simulink library "lib_dGrid"  (R2023b)
settings: Solver=VariableStepAuto  StartTime=0.0  StopTime=10.0  RelTol=1e-3
values from neighbouring files (symbols this model uses):
  C_PM = 10e-3    (= 0.01)    [my_MMC_param.m]
  Cbase = 1/Zbase/wb    (= 3.10849498226e-05)    [my_MMC_param.m]
  f0 = 50/fb    (= 1)    [my_MMC_param.m]
  Fn_filter = 1000    [my_MMC_param.m]
  Fnom = 50    [my_MMC_param.m]
  GFL_APC = 1    [Analysis_Main.m]    (also in initSimu.m; my_MMC_param.m)
  GFL_DVC = 2    [Analysis_Main.m]    (also in initSimu.m; my_MMC_param.m)
  GFM_APC = 3; (values programmed in EMT models)    [Analysis_Main.m]    (also in initSimu.m; my_MMC_param.m = 3)
  GFM_VF = 0    [my_MMC_param.m]
  Ibase = 2*Sbase/(3*Ubase)    [my_MMC_param.m]
  Idcb = Sbase/Udcb    [my_MMC_param.m]
  Ki_Iccsc = 5.15    [my_MMC_param.m]
  Ki_Ireg = CCCTRL.CC.ki    [my_MMC_param.m]
  Ki_Izscc = 100    [my_MMC_param.m]
  Ki_PLL = 1/(CCCTRL.PLL.v0*CCCTRL.PLL.T^2)    [my_MMC_param.m]
  Ki_Preg = 1.0*10    (= 10)    [my_MMC_param.m]
  Ki_Qreg = 1.0*10    (= 10)    [my_MMC_param.m]
  Ki_VAC_GFL = 50    [my_MMC_param.m]
  Ki_VACreg = 10    [my_MMC_param.m]
  Ki_VDCreg = 10    [my_MMC_param.m]
  Ki_WtReg = Kp_WtReg / 0.025    (= 1600)    [my_MMC_param.m]
  Kp_Iccsc = 0.21    [my_MMC_param.m]
  Kp_Ireg = CCCTRL.CC.kp    [my_MMC_param.m]
  Kp_Izscc = 10    [my_MMC_param.m]
  Kp_PLL = 2/CCCTRL.PLL.v0/CCCTRL.PLL.T    [my_MMC_param.m]
  Kp_Preg = 0.5/3*1    (= 0.166666666667)    [my_MMC_param.m]
  Kp_Qreg = 0.5/3*1    (= 0.166666666667)    [my_MMC_param.m]
  Kp_VAC_GFL = 0.5    [my_MMC_param.m]
  Kp_VACreg = 0.01    [my_MMC_param.m]
  Kp_VDCreg = 1    [my_MMC_param.m]
  Kp_WtReg = 40    [my_MMC_param.m]
  Kpv_GFM = 1    [my_MMC_param.m]
  Kpwm = 0.5    [my_MMC_param.m]
  Larm = Larm_pu*(Zbase/wb)    (= 0.0488923985178)    [my_MMC_param.m]
  Lff = Larm_pu/2    (= 0.075)    [my_MMC_param.m]
  Limits_Ireg = [ 2.0  -2.0]    [my_MMC_param.m]
  Limits_Preg = [ 2, -2 ]    [my_MMC_param.m]
  Limits_Qreg = 2*[ 0.42, -0.42 ]    [my_MMC_param.m]
  Limits_VACreg = [ 1.3  -1.3]    [my_MMC_param.m]
  Limits_VDCreg = [ 2.0  -2.0]    [my_MMC_param.m]
  MMC1 = MMC    [Analysis_Main.m]    (also in initSimu.m)
  Nb_PM = 400    [my_MMC_param.m]
  PhaseDelay = 1.0*Ts_Control*2*pi*50    (= 0.0628318530718)    [my_MMC_param.m]
  Pnom = 1000e6    (= 1000000000)    [my_MMC_param.m]
  Rarm = Rarm_pu*Zbase    (= 0.1536)    [my_MMC_param.m]
  Slope_Pref = 0.5    [my_MMC_param.m]
  Slope_Qref = 0.5    [my_MMC_param.m]
  Slope_Vdc_ref = Vnom_dc/2    (= 320000)    [my_MMC_param.m]
  Tdeblock = 1.5    [my_MMC_param.m]
  Ton_CROSSreg = Ton_PQreg+3    (= 7)    [my_MMC_param.m]
  Ton_PQreg = 4    [my_MMC_param.m]
  Ton_VDCreg = 1.5    [my_MMC_param.m]
  Ts = Ts_Control    (= 0.0002)    [my_MMC_param.m]
  Ts_Control = Ts_Power*2    (= 0.0002)    [my_MMC_param.m]
  Ts_Power = 20e-6 * 5    (= 0.0001)    [my_MMC_param.m]
  Ubase = sqrt(2/3)*Vnom_sec    [my_MMC_param.m]
  Udcb = 2*Ubase    [my_MMC_param.m]
  Vc0_PM = 0    [my_MMC_param.m]
  Vnom_dc = 640e3    (= 640000)    [my_MMC_param.m]
  Vnom_sec = 320e3    (= 320000)    [my_MMC_param.m]
  wb = 2*pi*fb    (= 314.159265359)    [my_MMC_param.m]
  Wt_ref_pu = 0.5 * C_PM * (Vnom_dc/Nb_PM)^2 * Nb_PM * 6 / Pnom    (= 0.03072)    [my_MMC_param.m]
undefined symbols (not defined in the file or in its folder): ControlSampleTime, DiscIntNeverNeededParam, MMC, PLL, VSM
libraries: simulink x50, spsCurrentMeasurementLib x20, spsSecondOrderFilterLib x20, spsDiodeLib x12, spsControlledVoltageSourceLib x12, spsSeriesRLCBranchLib x10, spsFirstOrderFilterLib x9, spsVoltageMeasurementLib x8, spsMeanLib x7, FriedrichLibrary x6, $bdroot x6, powerlib_extras x4
(part 7 of 8)

== system lib_dGrid/TL-VSC-configurable control modes/VSC Control/VF mode/PI regulator with anti-windup D1 ==
  note: Anti-windup mechanism: Method of conditionnal integration
      |
      | The integration is suspended if saturation occurs and the
      | control error is of the same sign as the control signal.
      |
      | [1] L.Rundqwist, "Anti-Reset Windup for PID Controllers," Ph.D. Thesis TRFT-1033,
      | Departement of Automatic Control, Lund Institute of Technology, Lund, Sweeden, 1991.
  Error : Inport  SampleTime=Ts
  Compare To Zero : simulink/Logic and Bit Operations/Compare To Zero  relop=>  OutDataTypeStr=uint8  ZeroCross=off
  Compare To Zero1 : simulink/Logic and Bit Operations/Compare To Zero  relop=<  OutDataTypeStr=uint8  ZeroCross=off
  Constant : Constant  Value=0
  Constant1 : Constant  Value=UpperLimit
  Constant3 : Constant  Value=LowerLimit
  Discrete-Time Integrator : DiscreteIntegrator  IntegratorMethod=Integration: Trapezoidal  InitialCondition=Init  SampleTime=Ts  LimitOutput=on  UpperSaturationLimit=UpperLimit  LowerSaturationLimit=LowerLimit  ShowStatePort=on  ICPrevOutput=DiscIntNeverNeededParam  ICPrevScaledInput=DiscIntNeverNeededParam
  Kp4 : Gain  Gain=Kp  SaturateOnIntegerOverflow=on  SampleTime=Ts  OutDataTypeStr=Inherit: Same as input  ParamDataTypeStr=Inherit: Same as input
  Kp5 : Gain  Gain=Ki  SaturateOnIntegerOverflow=on  SampleTime=Ts  OutDataTypeStr=Inherit: Same as input  ParamDataTypeStr=Inherit: Same as input
  Logical Operator : Logic  AllPortsSameDT=off  OutDataTypeStr=boolean
  Logical Operator1 : Logic  AllPortsSameDT=off  OutDataTypeStr=boolean
  Logical Operator2 : Logic  Operator=OR  AllPortsSameDT=off  OutDataTypeStr=boolean
  Relational Operator : RelationalOperator  OutDataTypeStr=boolean  InputSameDT=off
  Relational Operator1 : RelationalOperator  Operator=<=  OutDataTypeStr=boolean  InputSameDT=off
  Saturation2 : Saturate  UpperLimit=UpperLimit  LowerLimit=LowerLimit  SampleTime=Ts
  Sum1 : Sum  InputSameDT=on  SaturateOnIntegerOverflow=on  SampleTime=Ts  OutDataTypeStr=Inherit: Same as first input
  Sum6 : Sum  InputSameDT=on  SaturateOnIntegerOverflow=on  SampleTime=Ts  OutDataTypeStr=Inherit: Same as first input
  Switch : Switch  Criteria=u2 > Threshold  SaturateOnIntegerOverflow=off  InputSameDT=off
  Zero-Order Hold : ZeroOrderHold  SampleTime=Ts
  Out : Outport  SampleTime=Ts  InitialOutput=0  VectorParamsAs1DForOutWhenUnconnected=off
  wires:
  Kp5/1 -> Switch/3
  Switch/1 -> Discrete-Time Integrator/1
  Saturation2/1 -> Out/1
  Discrete-Time Integrator/1 -> Sum6/2
  Kp4/1 -> Zero-Order Hold/1
  Sum6/1 -> Saturation2/1
  Error/1 -> Kp5/1, Kp4/1, Compare To Zero/1, Compare To Zero1/1
  Compare To Zero1/1 -> Logical Operator1/2  "Error_is_negative"
  Logical Operator1/1 -> Logical Operator2/2
  Logical Operator/1 -> Logical Operator2/1
  Compare To Zero/1 -> Logical Operator/2  "Error_is_positive"
  Constant3/1 -> Relational Operator1/2
  Constant1/1 -> Relational Operator/2
  Relational Operator1/1 -> Logical Operator1/1  "LowerLimit_Is_Reached"
  Relational Operator/1 -> Logical Operator/1  "UpperLimit_is_Reached"
  Logical Operator2/1 -> Switch/2
  Sum1/1 -> Relational Operator/1, Relational Operator1/1
  Discrete-Time Integrator/State -> Sum1/1
  Zero-Order Hold/1 -> Sum6/1, Sum1/2
  Constant/1 -> Switch/1

== system lib_dGrid/TL-VSC-configurable control modes/VSC Control/VF mode/PI regulator with anti-windup D2 ==
  note: Anti-windup mechanism: Method of conditionnal integration
      |
      | The integration is suspended if saturation occurs and the
      | control error is of the same sign as the control signal.
      |
      | [1] L.Rundqwist, "Anti-Reset Windup for PID Controllers," Ph.D. Thesis TRFT-1033,
      | Departement of Automatic Control, Lund Institute of Technology, Lund, Sweeden, 1991.
  Error : Inport  SampleTime=Ts
  Compare To Zero : simulink/Logic and Bit Operations/Compare To Zero  relop=>  OutDataTypeStr=uint8  ZeroCross=off
  Compare To Zero1 : simulink/Logic and Bit Operations/Compare To Zero  relop=<  OutDataTypeStr=uint8  ZeroCross=off
  Constant : Constant  Value=0
  Constant1 : Constant  Value=UpperLimit
  Constant3 : Constant  Value=LowerLimit
  Discrete-Time Integrator : DiscreteIntegrator  IntegratorMethod=Integration: Trapezoidal  InitialCondition=Init  SampleTime=Ts  LimitOutput=on  UpperSaturationLimit=UpperLimit  LowerSaturationLimit=LowerLimit  ShowStatePort=on  ICPrevOutput=DiscIntNeverNeededParam  ICPrevScaledInput=DiscIntNeverNeededParam
  Kp4 : Gain  Gain=Kp  SaturateOnIntegerOverflow=on  SampleTime=Ts  OutDataTypeStr=Inherit: Same as input  ParamDataTypeStr=Inherit: Same as input
  Kp5 : Gain  Gain=Ki  SaturateOnIntegerOverflow=on  SampleTime=Ts  OutDataTypeStr=Inherit: Same as input  ParamDataTypeStr=Inherit: Same as input
  Logical Operator : Logic  AllPortsSameDT=off  OutDataTypeStr=boolean
  Logical Operator1 : Logic  AllPortsSameDT=off  OutDataTypeStr=boolean
  Logical Operator2 : Logic  Operator=OR  AllPortsSameDT=off  OutDataTypeStr=boolean
  Relational Operator : RelationalOperator  OutDataTypeStr=boolean  InputSameDT=off
  Relational Operator1 : RelationalOperator  Operator=<=  OutDataTypeStr=boolean  InputSameDT=off
  Saturation2 : Saturate  UpperLimit=UpperLimit  LowerLimit=LowerLimit  SampleTime=Ts
  Sum1 : Sum  InputSameDT=on  SaturateOnIntegerOverflow=on  SampleTime=Ts  OutDataTypeStr=Inherit: Same as first input
  Sum6 : Sum  InputSameDT=on  SaturateOnIntegerOverflow=on  SampleTime=Ts  OutDataTypeStr=Inherit: Same as first input
  Switch : Switch  Criteria=u2 > Threshold  SaturateOnIntegerOverflow=off  InputSameDT=off
  Zero-Order Hold : ZeroOrderHold  SampleTime=Ts
  Out : Outport  SampleTime=Ts  InitialOutput=0  VectorParamsAs1DForOutWhenUnconnected=off
  wires:
  Kp5/1 -> Switch/3
  Switch/1 -> Discrete-Time Integrator/1
  Saturation2/1 -> Out/1
  Discrete-Time Integrator/1 -> Sum6/2
  Kp4/1 -> Zero-Order Hold/1
  Sum6/1 -> Saturation2/1
  Error/1 -> Kp5/1, Kp4/1, Compare To Zero/1, Compare To Zero1/1
  Compare To Zero1/1 -> Logical Operator1/2  "Error_is_negative"
  Logical Operator1/1 -> Logical Operator2/2
  Logical Operator/1 -> Logical Operator2/1
  Compare To Zero/1 -> Logical Operator/2  "Error_is_positive"
  Constant3/1 -> Relational Operator1/2
  Constant1/1 -> Relational Operator/2
  Relational Operator1/1 -> Logical Operator1/1  "LowerLimit_Is_Reached"
  Relational Operator/1 -> Logical Operator/1  "UpperLimit_is_Reached"
  Logical Operator2/1 -> Switch/2
  Sum1/1 -> Relational Operator/1, Relational Operator1/1
  Discrete-Time Integrator/State -> Sum1/1
  Zero-Order Hold/1 -> Sum6/1, Sum1/2
  Constant/1 -> Switch/1

== system lib_dGrid/TL-VSC-configurable control modes/VSC Control/VSM Control/DQ damping1 Need New paras or New implementation ==
  enable_damp_dq : Inport
  u_dq0 : Inport  Port=2
  Gain2 : Gain  Gain=OmLead
  Gain5 : Gain  Gain=OmLag
  Integrator (inertia) : DiscreteIntegrator  IntegratorMethod=Integration: Backward Euler  gainval=1  InitialCondition=1  SampleTime=ControlSampleTime  ICPrevOutput=DiscIntNeverNeededParam  ICPrevScaledInput=DiscIntNeverNeededParam
  Product : Product
  Product1 : Product
  Sum : Sum  Inputs=|+-
  Sum2 : Sum  Inputs=++|
  Zero-Order Hold : ZeroOrderHold  SampleTime=Ts
  damp_dq0 : Outport  VectorParamsAs1DForOutWhenUnconnected=off
  wires:
  Product1/1 -> damp_dq0/1
  enable_damp_dq/1 -> Product1/1, Product/1
  Product/1 -> Gain2/1, Zero-Order Hold/1
  u_dq0/1 -> Product/2
  Sum/1 -> Integrator (inertia)/1
  Sum2/1 -> Gain5/1, Product1/2
  Gain5/1 -> Sum/2
  Integrator (inertia)/1 -> Sum2/2
  Gain2/1 -> Sum/1
  Zero-Order Hold/1 -> Sum2/1

== system lib_dGrid/TL-VSC-configurable control modes/VSC Control/VSM Control/Inner Loop Control ==
  IdIq : Inport  PortDimensions=2
  In : Inport  Port=2
  VdVq : Inport  Port=3  PortDimensions=2
  Enable : EnablePort  StatesWhenEnabling=reset
  1st-Order LPF : spsFirstOrderFilterLib/First-Order Filter  Commented=through  FilterType=Lowpass  Tc=1/(2*pi*Fn_filter/10)  Ts=Ts  Initialize=on  Vac_Init=[0, 0, 50]  Vdc_Init=0  PlotResponse=off  FreqRange="[0,  200,  1]"
  CC : Subsystem  DialogController=POWERSYS.PowerSysDialog  mask(Discrete PI Controller){Kp=Kp_Ireg, Ki=Ki_Ireg, Par_Limits=Limits_Ireg, Init=0, Ts=Ts_Control}
      mask prompts: Kp "Proportional gain (Kp):"; Ki "Integral gain (Ki):"; Par_Limits "Output limits: [ Upper   Lower ]"; Init "Output initial value:"; Ts "Sample time:"
      mask help: This block implements a discrete PI controller.
      mask init:
      | UpperLimit=Par_Limits(1);
      | LowerLimit=Par_Limits(2);
      | power_initmask();
      mask Help: This block is part of a subset of blocks in the Extras library that does not have documentation associated with it, other than the block mask description.
      mask Display: disp('PI');
  "CC " : Subsystem  DialogController=POWERSYS.PowerSysDialog  mask(Discrete PI Controller){Kp=Kp_Ireg, Ki=Ki_Ireg, Par_Limits=Limits_Ireg, Init=0, Ts=Ts_Control}
      mask prompts: Kp "Proportional gain (Kp):"; Ki "Integral gain (Ki):"; Par_Limits "Output limits: [ Upper   Lower ]"; Init "Output initial value:"; Ts "Sample time:"
      mask help: This block implements a discrete PI controller.
      mask init:
      | UpperLimit=Par_Limits(1);
      | LowerLimit=Par_Limits(2);
      | power_initmask();
      mask Help: This block is part of a subset of blocks in the Extras library that does not have documentation associated with it, other than the block mask description.
      mask Display: disp('PI');
  Cartesian to Polar1 : simulink_extras/Transformations/Cartesian to Polar
  Constant5 : Constant  Value=Lff  SampleTime=Ts_Control
  Constant6 : Constant  Value=Lff  SampleTime=Ts_Control
  Demux1 : Demux  Outputs=2
  Demux2 : Demux  Outputs=2
  Demux3 : Demux  Outputs=2
  Gain1 : Gain  Gain=Kpv_GFM
  Gain{2..3,5..6} (4 alike) : Gain
  Kpv_GFM : Gain  Gain=Kpv_GFM
  Mux3 : Mux  Inputs=2
  Polar to Cartesian : simulink_extras/Transformations/Polar to Cartesian
  Product3 : Product  RndMeth=Zero
  Product4 : Product  RndMeth=Zero
  Saturation1 : Saturate  UpperLimit=1.2  LowerLimit=-1.2
  Sum1 : Sum  Inputs=++|
  Sum2 : Sum  Inputs=-+|
  Sum3 : Sum  Inputs=|+-
  Sum4 : Sum  Inputs=+-+|
  Sum5 : Sum  Inputs=|+++
  Sum6 : Sum  Inputs=|++
  Sum7 : Sum  Inputs=-+|
  Sum8 : Sum  Inputs=|+-
  Out : Outport
  wires:
  Product4/1 -> Gain5/1
  Sum2/1 -> Gain1/1
  Constant6/1 -> Product3/2
  Saturation1/1 -> Polar to Cartesian/1
  In/1 -> Demux1/1
  Sum4/1 -> Mux3/1
  Sum3/1 -> Kpv_GFM/1
  Demux1/1 -> Sum2/2
  Product3/1 -> Gain6/1
  Demux1/2 -> Sum3/1
  [Id] -> Sum7/1, Sum1/1
  Constant5/1 -> Product4/2
  "CC "/1(Out) -> Sum5/1
  Sum5/1 -> Mux3/2
  [Vd] -> Sum2/1, Gain2/1
  Polar to Cartesian/2 -> Sum8/1
  [Iq] -> Sum8/2, Sum6/2
  CC/1(Out) -> Sum4/3
  Gain2/1 -> Sum4/1
  Sum1/1 -> Cartesian to Polar1/1
  [Iq] -> Product3/1
  Cartesian to Polar1/1 -> [Im_ref], Saturation1/1
  Sum7/1 -> CC/1(Error)
  Gain6/1 -> Sum4/2
  Gain1/1 -> Sum1/2
  [Vq] -> Gain3/1, Sum3/2
  Cartesian to Polar1/2 -> Polar to Cartesian/2
  [Id] -> Product4/1
  Kpv_GFM/1 -> Sum6/1
  Polar to Cartesian/1 -> Sum7/2
  Sum6/1 -> Cartesian to Polar1/2
  Gain3/1 -> Sum5/3
  Gain5/1 -> Sum5/2
  Sum8/1 -> "CC "/1(Error)
  VdVq/1 -> 1st-Order LPF/1
  Demux3/2 -> [Vq]
  Demux3/1 -> [Vd]
  IdIq/1 -> Demux2/1
  Demux2/2 -> [Iq]
  Demux2/1 -> [Id]
  Mux3/1 -> Out/1
  1st-Order LPF/1 -> Demux3/1

== system lib_dGrid/TL-VSC-configurable control modes/VSC Control/VSM Control/Modulation Gain ==
  note: Original implementation for modulation compensation
      |
      |
      |
      |
      |
      |
      |
      |
      | Equivalent to the control output divided by Vdc_pu
      | which can be calculated by Vdc/Vdc_base
      | where Vdc_base = 2 * Vbase with
      | Vbase = sqrt(2)/sqrt(3)*Vnom_sec
  Uref : Inport
  " (Hz)" : Constant  Commented=on  Value=Vnom_dc  SampleTime=Ts
  " (Hz)1" : Constant  Value=Vnom_dc  SampleTime=Ts
  ->pu : Gain  Gain=1/Udcb
  Avoid division by zero1 : Saturate  Commented=on  UpperLimit=Vnom_dc*1.25  LowerLimit=Vnom_dc*0.75
  Avoid division by zero2 : Saturate  UpperLimit=Vnom_dc*1.25  LowerLimit=Vnom_dc*0.75
  Divide : Product  Commented=on  Inputs=*/
  Divide1 : Product  Commented=on  Inputs=**
  Divide2 : Product  Inputs=*/
  Mean : spsMeanLib/Mean  Commented=on  Freq=Fnom/3  Vinit=Vnom_dc  Ts=Ts
  to-pu : Gain  Commented=on  Gain=1/(Vnom_dc/2*sqrt(3)/sqrt(2)/Vnom_sec)
  out : Outport
  wires:
  Divide1/1 -> to-pu/1
  " (Hz)"/1 -> Divide/1
  Divide/1 -> Divide1/2
  Divide2/1 -> out/1
  Avoid division by zero1/1 -> Divide/2
  ->pu/1 -> Divide2/2  "udc_pu"
  Uref/1 -> Divide2/1
  Avoid division by zero2/1 -> ->pu/1
  " (Hz)1"/1 -> Avoid division by zero2/1
  Mean/1 -> Avoid division by zero1/1

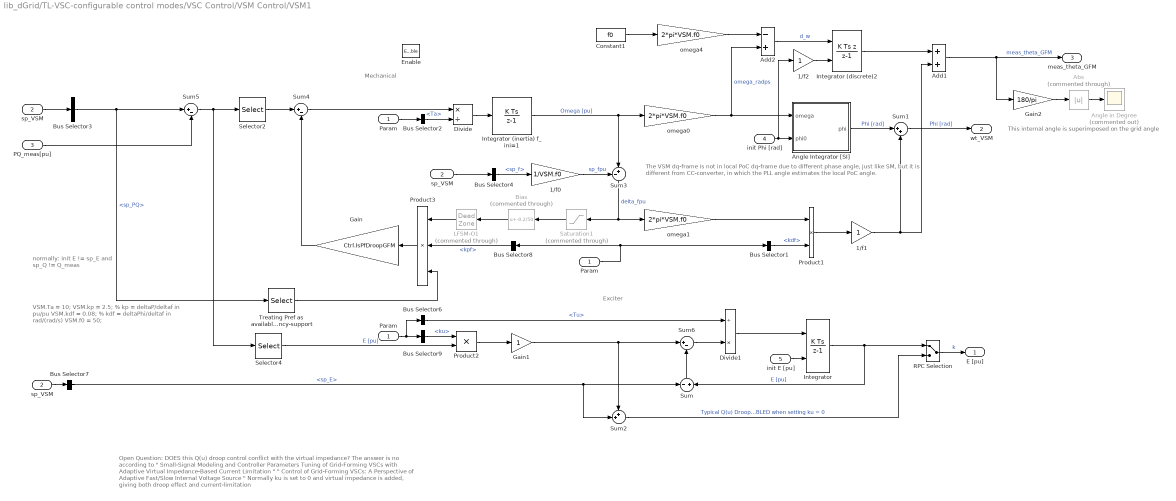
== system lib_dGrid/TL-VSC-configurable control modes/VSC Control/VSM Control/VSM1 ==
  note: This internal angle is superimposed
      | on the grid angle
  note: Open Question: DOES this Q(u) droop control conflict with the virtual impedance?
      | The answer is no according to
      | " Small-Signal Modeling and Controller Parameters Tuning of Grid-Forming VSCs with Adaptive Virtual Impedance-Based Current Limitation "
      | " Control of Grid-Forming VSCs: A Perspective of Adaptive Fast/Slow Internal Voltage Source "
      | Normally ku is set to 0 and virtual impedance is added, giving both droop effect and current-limitation
  note: The VSM dq-frame is not in local PoC dq-frame due to different phase angle, just like SM, but it is different from CC-converter, in which the PLL angle estimates the local PoC angle.
  note: Exciter
  note: VSM.Ta = 10;
      | VSM.kp = 2.5; % kp = deltaP/deltaf  in  pu/pu
      | VSM.kdf = 0.08; % kdf = deltaPhi/deltaf in rad/(rad/s)
      | VSM.f0 = 50;
  note: normally:
      | init E != sp_E
      | and
      | sp_Q != Q_meas
  note: Mechanical
  Param : Inport
  sp_VSM : Inport  Port=2
  PQ_meas[pu] : Inport  Port=3
  init Phi [rad] : Inport  Port=4
  init E [pu] : Inport  Port=5
  Enable : EnablePort  StatesWhenEnabling=reset
  " Param " : InportShadow
  " sp_VSM " : InportShadow  Port=2
  1/f0 : Gain  Gain=1/VSM.f0
  1/f1 : Gain
  1/f2 : Gain
  Abs : Abs  Commented=through  SaturateOnIntegerOverflow=off
  Add1 : Sum
  Add2 : Sum  Inputs=-+
  Angle Integrator [SI] : Subsystem  AncestorBlock=FriedrichLibrary/Discrete Stuff/Angle Integrator [SI]  mask{Ts=Ts_Control}
      mask prompts: Ts "SampleTime"
      mask DialogControl DescGroupVar Prompt: Angle Integrator [SI]
      mask DialogControl DescTextVar Prompt: Discrete Integrator for omega, resetting every 2*pi.
  Angle in Degree : Scope  Commented=on
  Bias : Bias  Commented=through  Bias=-0.2/50  SaturateOnIntegerOverflow=off
  Bus Selector1 : BusSelector  OutputSignals=kdf
  Bus Selector2 : BusSelector  OutputSignals=Ta
  Bus Selector3 : BusSelector  OutputSignals=sp_PQ
  Bus Selector4 : BusSelector  OutputSignals=sp_f
  Bus Selector6 : BusSelector  OutputSignals=Tu
  Bus Selector7 : BusSelector  OutputSignals=sp_E
  Bus Selector8 : BusSelector  OutputSignals=kpf
  Bus Selector9 : BusSelector  OutputSignals=ku
  Constant1 : Constant  Value=f0
  Divide : Product  Inputs=*/
  Divide1 : Product  Inputs=/*
  Gain : Gain  Gain=Ctrl.IsPfDroopGFM
  Gain1 : Gain
  Gain2 : Gain  Gain=180/pi
  Integrator : DiscreteIntegrator  gainval=1  InitialConditionSource=external  InitialCondition=0.9  SampleTime=Ts_Control  ICPrevOutput=DiscIntNeverNeededParam  ICPrevScaledInput=DiscIntNeverNeededParam
  Integrator (discrete)2 : DiscreteIntegrator  IntegratorMethod=Integration: Backward Euler  gainval=1  InitialConditionSource=external  SampleTime=Ts_Control  ICPrevOutput=DiscIntNeverNeededParam  ICPrevScaledInput=DiscIntNeverNeededParam
  Integrator (inertia) f_ini=1 : DiscreteIntegrator  gainval=1  InitialCondition=1  SampleTime=Ts_Control  ICPrevOutput=DiscIntNeverNeededParam  ICPrevScaledInput=DiscIntNeverNeededParam
  LFSM-O1 : DeadZone  Commented=through  LowerValue=-VSM.IPF.Deadband*1e6  UpperValue=VSM.IPF.Deadband
  "Param " : InportShadow
  Product1 : Product
  Product2 : Product
  Product3 : Product  Inputs=3
  RPC Selection : ManualSwitch
  Saturation1 : Saturate  Commented=through  UpperLimit=Inf  LowerLimit=0.2/50
  Selector2 : Selector  InputPortWidth=2  IndexOptions=Index vector (dialog)  Indices=1  OutputSizes=1
  Selector4 : Selector  InputPortWidth=2  IndexOptions=Index vector (dialog)  Indices=2  OutputSizes=1
  Sum : Sum  Inputs=-|+
  Sum1 : Sum  Inputs=|++
  Sum2 : Sum  Inputs=++|
  Sum3 : Sum  Inputs=-+|
  Sum4 : Sum  Inputs=|+-
  Sum5 : Sum  Inputs=|+-
  Sum6 : Sum  Inputs=|+-
  Treating Pref as available mechanical Power that is used for frequency-support : Selector  InputPortWidth=2  IndexOptions=Index vector (dialog)  Indices=1  OutputSizes=1
  omega0 : Gain  Gain=2*pi*VSM.f0
  omega1 : Gain  Gain=2*pi*VSM.f0
  omega4 : Gain  Gain=2*pi*VSM.f0
  "sp_VSM " : InportShadow  Port=2
  E [pu] : Outport  VectorParamsAs1DForOutWhenUnconnected=off
  wt_VSM : Outport  Port=2  VectorParamsAs1DForOutWhenUnconnected=off
  meas_theta_GFM : Outport  Port=3  VectorParamsAs1DForOutWhenUnconnected=off
  wires:
  Integrator (inertia) f_ini=1/1 -> omega0/1, Sum3/2  "Omega [pu]"
  Product3/1 -> Gain/1
  Sum4/1 -> Divide/1
  Product1/1 -> 1/f1/1
  Angle Integrator [SI]/1(phi) -> Sum1/1  "Phi [rad]"
  Sum3/1 -> Saturation1/1, omega1/1  "delta_fpu"
  Bus Selector4/1 -> 1/f0/1  "<sp_f>"
  Param/1 -> Bus Selector2/1
  "Param "/1 -> Bus Selector1/1, Bus Selector8/1
  Bus Selector8/1 -> Product3/2  "<kpf>"
  Bus Selector1/1 -> Product1/2  "<kdf>"
  omega0/1 -> Angle Integrator [SI]/1(omega), Add2/2  "omega_radps"
  "sp_VSM "/1 -> Bus Selector4/1
  1/f0/1 -> Sum3/1  "sp_fpu"
  Integrator/1 -> RPC Selection/1, Sum/2  "E [pu]"
  Divide1/1 -> Integrator/1
  Sum6/1 -> Divide1/2
  Bus Selector6/1 -> Divide1/1  "<Tu>"
  " sp_VSM "/1 -> Bus Selector7/1
  Bus Selector7/1 -> Sum2/2, Sum/1  "<sp_E>"
  init E [pu]/1 -> Integrator/2
  omega1/1 -> Product1/1
  Selector2/1 -> Sum4/1
  Sum/1 -> Sum6/2
  Bus Selector2/1 -> Divide/2  "<Ta>"
  sp_VSM/1 -> Bus Selector3/1
  Sum5/1 -> Selector4/1, Selector2/1
  " Param "/1 -> Bus Selector6/1, Bus Selector9/1
  Bus Selector9/1 -> Product2/1  "<ku>"
  Sum1/1 -> wt_VSM/1  "Phi [rad]"
  1/f1/1 -> Sum1/2, Add1/2
  init Phi [rad]/1 -> Angle Integrator [SI]/2(phi0), 1/f2/1
  Divide/1 -> Integrator (inertia) f_ini=1/1
  Saturation1/1 -> Bias/1
  LFSM-O1/1 -> Product3/1
  Bias/1 -> LFSM-O1/1
  1/f2/1 -> Integrator (discrete)2/2
  Add2/1 -> Integrator (discrete)2/1  "d_w"
  Constant1/1 -> omega4/1
  Add1/1 -> meas_theta_GFM/1, Gain2/1  "meas_theta_GFM"
  Integrator (discrete)2/1 -> Add1/1
  omega4/1 -> Add2/1
  Bus Selector3/1 -> Sum5/1, Treating Pref as available mechanical Power that is used for frequency-support/1  "<sp_PQ>"
  Treating Pref as available mechanical Power that is used for frequency-support/1 -> Product3/3
  Gain/1 -> Sum4/2
  PQ_meas[pu]/1 -> Sum5/2
  Product2/1 -> Gain1/1
  Sum2/1 -> RPC Selection/2  "Typical Q(u) Droop Control  with Q passing through a LPF in the Measurement Block The other control option has Tu and T_LPF two time constants if Q has LPF - Q(u) droop is DISABLED when setting ku = 0"
  RPC Selection/1 -> E [pu]/1  "k"
  Gain1/1 -> Sum6/1, Sum2/1
  Selector4/1 -> Product2/2  "E [pu]"
  Abs/1 -> Angle in Degree/1
  Gain2/1 -> Abs/1

== system lib_dGrid/TL-VSC-configurable control modes/VSC Control/VSM Control/Virtual circuit daniel style1 ==
  i_dq : Inport
  Add1 : Sum  Inputs=+-
  Add2 : Sum
  Constant : Constant  Value=VSM.VC.rv
  Constant1 : Constant  Value=VSM.VC.xv
  Demux : Demux  Outputs=2
  Mux : Mux  Inputs=2
  Product{1..4} (4 alike) : Product
  transient rv (HP)1 -dd's form : Subsystem  mask{TS=Ts_Control, tau=VSM.VC.tau_rv}
      mask prompts: TS "sample time"; tau "high pass time constant"
  transient rv (HP)1 yz's form : Subsystem  Commented=on  mask{TS=ControlSampleTime, tau=VSM.VC.tau_rv}
      mask prompts: TS "sample time"; tau "high pass time constant"
  transient rv (HP)2 (dd's form) : Subsystem  mask{TS=Ts_Control, tau=VSM.VC.tau_rv}
      mask prompts: TS "sample time"; tau "high pass time constant"
  v_vc_dq : Outport  VectorParamsAs1DForOutWhenUnconnected=off
  wires:
  transient rv (HP)2 (dd's form)/1(Out1) -> Add2/2
  Demux/2 -> Product2/2, Product3/1
  Add2/1 -> Mux/2
  Product3/1 -> Add1/2
  Add1/1 -> Mux/1
  transient rv (HP)1 -dd's form/1(Out1) -> Add1/1
  Product1/1 -> transient rv (HP)1 -dd's form/1(In1)
  Product2/1 -> transient rv (HP)2 (dd's form)/1(In1)
  Mux/1 -> v_vc_dq/1
  i_dq/1 -> Demux/1
  Constant/1 -> Product2/1, Product1/2
  Constant1/1 -> Product4/1, Product3/2
  Product4/1 -> Add2/1
  Demux/1 -> Product1/1, Product4/2

== system lib_dGrid/TL-VSC-configurable control modes/VSC Control/VSM Control/cmd_VSM ==
  Pref : Inport  PortDimensions=1
  Qref : Inport  Port=2  PortDimensions=1
  Bus Creator1 : BusCreator  Inputs=1
  Bus Creator3 : BusCreator  Inputs=7
  Bus Creator4 : BusCreator  Inputs=3
  Bus Creator15 : BusCreator  Inputs=5
  Constant : Constant
  Constant1 : Constant
  Constant4 : Constant
  EnableDamp_CM [0/1] : Constant  Value=0
  EnableDamp_dq [0/1] : Constant
  Mux : Mux  Inputs=2
  "Set Eref to 1 when adopting Q(U) droop " : Constant  Value=1.0
  Ta : Constant  Value=VSM.Ta
  Ta1 : Constant  Value=VSM.kpf
  Ta2 : Constant  Value=VSM.kdf
  Ta3 : Constant  Value=VSM.ku
  Ta4 : Constant  Value=VSM.Tu
  sp_f [Hz] : Constant  Value=50
  cmd_ac : Outport  VectorParamsAs1DForOutWhenUnconnected=off
  wires:
  Bus Creator15/1 -> cmd_ac/1
  Constant4/1 -> Bus Creator15/2  "connect"
  Constant/1 -> Bus Creator15/1  "preload"
  Bus Creator1/1 -> Bus Creator15/5  "Param"
  Constant1/1 -> Bus Creator15/3  "enable"
  Ta/1 -> Bus Creator3/1  "Ta"
  Bus Creator3/1 -> Bus Creator1/1  "VSM"
  Ta2/1 -> Bus Creator3/3  "kdf"
  Ta1/1 -> Bus Creator3/2  "kpf"
  Ta3/1 -> Bus Creator3/4  "ku"
  Ta4/1 -> Bus Creator3/5  "Tu"
  Bus Creator4/1 -> Bus Creator15/4  "sp_VSM"
  sp_f [Hz]/1 -> Bus Creator4/1  "sp_f"
  Mux/1 -> Bus Creator4/2  "sp_PQ"
  "Set Eref to 1 when adopting Q(U) droop "/1 -> Bus Creator4/3  "sp_E"
  EnableDamp_dq [0/1]/1 -> Bus Creator3/6  "EnableDamp_dq"
  EnableDamp_CM [0/1]/1 -> Bus Creator3/7  "EnableDamp_CM"
  Qref/1 -> Mux/2
  Pref/1 -> Mux/1

== system lib_dGrid/MMC-configurable control modes/MMC Control/CCSC + ZSCC control/PR control/PR Controller ==
  In1 : Inport
  Gain : Gain  Gain=kp
  Gain1 : Gain  Gain=kr
  Sum1 : Sum  Inputs=|++
  Transfer Fcn1 : TransferFcn  Numerator=[1 0]  Denominator=[1 0 (2*pi*f)^2]
  Out1 : Outport
  wires:
  Gain1/1 -> Transfer Fcn1/1
  Transfer Fcn1/1 -> Sum1/2
  In1/1 -> Gain1/1, Gain/1
  Sum1/1 -> Out1/1
  Gain/1 -> Sum1/1

== system lib_dGrid/MMC-configurable control modes/MMC Control/CCSC + ZSCC control/PR control/PR Controller1 ==
  In1 : Inport
  Gain : Gain  Gain=kp
  Gain1 : Gain  Gain=kr
  Sum1 : Sum  Inputs=|++
  Transfer Fcn1 : TransferFcn  Numerator=[1 0]  Denominator=[1 0 (2*pi*f)^2]
  Out1 : Outport
  wires:
  Gain1/1 -> Transfer Fcn1/1
  Transfer Fcn1/1 -> Sum1/2
  In1/1 -> Gain1/1, Gain/1
  Sum1/1 -> Out1/1
  Gain/1 -> Sum1/1

== system lib_dGrid/MMC-configurable control modes/MMC Control/CCSC + ZSCC control/PR control/PR Controller2 ==
  In1 : Inport
  Gain : Gain  Gain=kp
  Gain1 : Gain  Gain=kr
  Sum1 : Sum  Inputs=|++
  Transfer Fcn1 : TransferFcn  Numerator=[1 0]  Denominator=[1 0 (2*pi*f)^2]
  Out1 : Outport
  wires:
  Gain1/1 -> Transfer Fcn1/1
  Transfer Fcn1/1 -> Sum1/2
  In1/1 -> Gain1/1, Gain/1
  Sum1/1 -> Out1/1
  Gain/1 -> Sum1/1

== system lib_dGrid/MMC-configurable control modes/MMC Control/CCSC + ZSCC control/Subsystem/EnergyCalc ==
  wt : Inport
  Uc_sum : Inport  Port=2
  Uc_diff : Inport  Port=3
  Add : Sum
  Add1 : Sum
  Constant2 : Constant  Commented=on  Value=90
  Demux : Demux  Outputs=2
  Demux2 : Demux  Outputs=2
  Display{,1..7} (8 alike) : Display  Commented=on
  Gain : Gain
  Gain1 : Gain  Gain=-2
  Gain2 : Gain
  Note that for p.u. representation: Epu = 0.5 * Cpu / wb * Upu^2 : Gain  Gain=1 / 2 * C_PM/Cbase / Nb_PM / wb
  PhN->ab2 : Subsystem  AncestorBlock=FriedrichLibrary/Transformations/PhN->ab0
      mask Display:
      | plot([0 1], [0,1])
      | plot([0.1 0.25 0.4 0.25 0.25], [0.5 0.6 0.5 0.6 0.8]) % Stern
      | text(0.05,1,'PhN','VerticalAlignment','Top')
      | text(0.55, 0.3,'\alpha\beta0','texmode','on')
  Plus1 : Sum  Inputs=+++
  Selector1 : Selector  InputPortWidth=3  IndexOptions=Index vector (dialog)  Indices=3  OutputSizes=1
  Selector2 : Selector  InputPortWidth=3  IndexOptions=Index vector (dialog)  Indices=[1 2]  OutputSizes=1
  Selector3 : Selector  InputPortWidth=3  IndexOptions=Index vector (dialog)  Indices=[1 2]  OutputSizes=1
  Sequence Analyzer2 : spsSequenceAnalyzerLib/Sequence Analyzer  Commented=on  Freq=50  n=1  seq=Positive Negative Zero  InInit=[1, 0]  Ts=Ts_Power
      settings: LibrarySourceBlock=sps_lib/Sensors and Measurements/Sequence Analyzer
  Square{,1..4} (5 alike) : Math  Operator=square
  Sum1 : Sum  Commented=on  Inputs=|+-
  Why this gain in literature??? : Gain  Commented=through  Gain=2
  ab0->dq0-faster1 : Subsystem  AncestorBlock=FriedrichLibrary/Transformations/ab0->dq0-faster
      mask Display:
      | plot([0 1], [0,1])
      | text(0.05,0.8,'\alpha\beta0','texmode','on')
      | text(1, 0.5,'dq0','HorizontalAlignment','right')
      | text(0.05,0.3,'\phi','texmode','on')
  abc to +1dq : spsabctodq0Lib/abc to dq0  Alignment=Aligned with phase A axis
  Wt in pu : Outport
  wires:
  abc to +1dq/1 -> Display5/1, Selector3/1
  Demux/1 -> Square1/1
  Uc_sum/1 -> PhN->ab2/1(PhN)
  Add1/1 -> Gain2/1
  Demux/2 -> Square2/1
  ab0->dq0-faster1/1(dq0) -> Display3/1, Selector2/1
  wt/1 -> Gain1/1, abc to +1dq/2
  Selector3/1 -> Demux2/1
  Demux2/1 -> Square3/1
  Demux2/2 -> Square4/1
  Add/1 -> Gain/1
  Selector2/1 -> Demux/1
  Plus1/1 -> Note that for p.u. representation: Epu = 0.5 * Cpu / wb * Upu^2/1
  Gain1/1 -> ab0->dq0-faster1/2(w)
  Note that for p.u. representation: Epu = 0.5 * Cpu / wb * Upu^2/1 -> Wt in pu/1
  PhN->ab2/1(ab0) -> Selector1/1, ab0->dq0-faster1/1(ab0)
  Selector1/1 -> Display4/1, Square/1  "meas_Uc_sum_z"
  Square/1 -> Why this gain in literature???/1
  Why this gain in literature???/1 -> Display1/1, Plus1/2
  Uc_diff/1 -> Sequence Analyzer2/1, abc to +1dq/1
  Sum1/1 -> Display7/1  "phase_pnz"
  Constant2/1 -> Sum1/2
  Sequence Analyzer2/2 -> Sum1/1
  Sequence Analyzer2/1 -> Display6/1  "mag_pnz"
  Gain/1 -> Display/1, Plus1/1
  Gain2/1 -> Display2/1, Plus1/3
  Square1/1 -> Add/1
  Square2/1 -> Add/2
  Square4/1 -> Add1/2
  Square3/1 -> Add1/1

== system lib_dGrid/MMC-configurable control modes/MMC Control/CCSC + ZSCC control/Subsystem/PI regulator with anti-windup D4 ==
  note: Anti-windup mechanism: Method of conditionnal integration
      |
      | The integration is suspended if saturation occurs and the
      | control error is of the same sign as the control signal.
      |
      | [1] L.Rundqwist, "Anti-Reset Windup for PID Controllers," Ph.D. Thesis TRFT-1033,
      | Departement of Automatic Control, Lund Institute of Technology, Lund, Sweeden, 1991.
  Error : Inport  SampleTime=Ts
  Compare To Zero : simulink/Logic and Bit Operations/Compare To Zero  relop=>  OutDataTypeStr=uint8  ZeroCross=off
  Compare To Zero1 : simulink/Logic and Bit Operations/Compare To Zero  relop=<  OutDataTypeStr=uint8  ZeroCross=off
  Constant : Constant  Value=0
  Constant1 : Constant  Value=UpperLimit
  Constant3 : Constant  Value=LowerLimit
  Discrete-Time Integrator : DiscreteIntegrator  IntegratorMethod=Integration: Trapezoidal  InitialCondition=Init  SampleTime=Ts  LimitOutput=on  UpperSaturationLimit=UpperLimit  LowerSaturationLimit=LowerLimit  ShowStatePort=on  ICPrevOutput=DiscIntNeverNeededParam  ICPrevScaledInput=DiscIntNeverNeededParam
  Kp4 : Gain  Gain=Kp  SaturateOnIntegerOverflow=on  SampleTime=Ts  OutDataTypeStr=Inherit: Same as input  ParamDataTypeStr=Inherit: Same as input
  Kp5 : Gain  Gain=Ki  SaturateOnIntegerOverflow=on  SampleTime=Ts  OutDataTypeStr=Inherit: Same as input  ParamDataTypeStr=Inherit: Same as input
  Logical Operator : Logic  AllPortsSameDT=off  OutDataTypeStr=boolean
  Logical Operator1 : Logic  AllPortsSameDT=off  OutDataTypeStr=boolean
  Logical Operator2 : Logic  Operator=OR  AllPortsSameDT=off  OutDataTypeStr=boolean
  Relational Operator : RelationalOperator  OutDataTypeStr=boolean  InputSameDT=off
  Relational Operator1 : RelationalOperator  Operator=<=  OutDataTypeStr=boolean  InputSameDT=off
  Saturation2 : Saturate  UpperLimit=UpperLimit  LowerLimit=LowerLimit  SampleTime=Ts
  Sum1 : Sum  InputSameDT=on  SaturateOnIntegerOverflow=on  SampleTime=Ts  OutDataTypeStr=Inherit: Same as first input
  Sum6 : Sum  InputSameDT=on  SaturateOnIntegerOverflow=on  SampleTime=Ts  OutDataTypeStr=Inherit: Same as first input
  Switch : Switch  Criteria=u2 > Threshold  SaturateOnIntegerOverflow=off  InputSameDT=off
  Zero-Order Hold : ZeroOrderHold  SampleTime=Ts
  Out : Outport  SampleTime=Ts  InitialOutput=0  VectorParamsAs1DForOutWhenUnconnected=off
  wires:
  Constant/1 -> Switch/1
  Zero-Order Hold/1 -> Sum1/2, Sum6/1
  Discrete-Time Integrator/State -> Sum1/1
  Sum1/1 -> Relational Operator1/1, Relational Operator/1
  Logical Operator2/1 -> Switch/2
  Relational Operator/1 -> Logical Operator/1  "UpperLimit_is_Reached"
  Relational Operator1/1 -> Logical Operator1/1  "LowerLimit_Is_Reached"
  Constant1/1 -> Relational Operator/2
  Constant3/1 -> Relational Operator1/2
  Compare To Zero/1 -> Logical Operator/2  "Error_is_positive"
  Logical Operator/1 -> Logical Operator2/1
  Logical Operator1/1 -> Logical Operator2/2
  Compare To Zero1/1 -> Logical Operator1/2  "Error_is_negative"
  Error/1 -> Compare To Zero1/1, Compare To Zero/1, Kp4/1, Kp5/1
  Sum6/1 -> Saturation2/1
  Kp4/1 -> Zero-Order Hold/1
  Discrete-Time Integrator/1 -> Sum6/2
  Saturation2/1 -> Out/1
  Switch/1 -> Discrete-Time Integrator/1
  Kp5/1 -> Switch/3

== system lib_dGrid/MMC-configurable control modes/MMC Control/CCSC + ZSCC control/Subsystem/PI with anti-windup ==
  note: Anti-windup mechanism: Method of conditionnal integration
      |
      | The integration is suspended if saturation occurs and the
      | control error is of the same sign as the control signal.
      |
      | [1] L.Rundqwist, "Anti-Reset Windup for PID Controllers," Ph.D. Thesis TRFT-1033,
      | Departement of Automatic Control, Lund Institute of Technology, Lund, Sweeden, 1991.
  Error : Inport  SampleTime=Ts
  Compare To Zero : simulink/Logic and Bit Operations/Compare To Zero  relop=>  OutDataTypeStr=uint8  ZeroCross=off
  Compare To Zero1 : simulink/Logic and Bit Operations/Compare To Zero  relop=<  OutDataTypeStr=uint8  ZeroCross=off
  Constant : Constant  Value=0
  Constant1 : Constant  Value=UpperLimit
  Constant3 : Constant  Value=LowerLimit
  Discrete-Time Integrator : DiscreteIntegrator  IntegratorMethod=Integration: Trapezoidal  InitialCondition=Init  SampleTime=Ts  LimitOutput=on  UpperSaturationLimit=UpperLimit  LowerSaturationLimit=LowerLimit  ShowStatePort=on  ICPrevOutput=DiscIntNeverNeededParam  ICPrevScaledInput=DiscIntNeverNeededParam
  Kp4 : Gain  Gain=Kp  SaturateOnIntegerOverflow=on  SampleTime=Ts  OutDataTypeStr=Inherit: Same as input  ParamDataTypeStr=Inherit: Same as input
  Kp5 : Gain  Gain=Ki  SaturateOnIntegerOverflow=on  SampleTime=Ts  OutDataTypeStr=Inherit: Same as input  ParamDataTypeStr=Inherit: Same as input
  Logical Operator : Logic  AllPortsSameDT=off  OutDataTypeStr=boolean
  Logical Operator1 : Logic  AllPortsSameDT=off  OutDataTypeStr=boolean
  Logical Operator2 : Logic  Operator=OR  AllPortsSameDT=off  OutDataTypeStr=boolean
  Relational Operator : RelationalOperator  OutDataTypeStr=boolean  InputSameDT=off
  Relational Operator1 : RelationalOperator  Operator=<=  OutDataTypeStr=boolean  InputSameDT=off
  Saturation2 : Saturate  UpperLimit=UpperLimit  LowerLimit=LowerLimit  SampleTime=Ts
  Sum1 : Sum  InputSameDT=on  SaturateOnIntegerOverflow=on  SampleTime=Ts  OutDataTypeStr=Inherit: Same as first input
  Sum6 : Sum  InputSameDT=on  SaturateOnIntegerOverflow=on  SampleTime=Ts  OutDataTypeStr=Inherit: Same as first input
  Switch : Switch  Criteria=u2 > Threshold  SaturateOnIntegerOverflow=off  InputSameDT=off
  Zero-Order Hold : ZeroOrderHold  SampleTime=Ts
  Out : Outport  SampleTime=Ts  InitialOutput=0  VectorParamsAs1DForOutWhenUnconnected=off
  wires:
  Constant/1 -> Switch/1
  Zero-Order Hold/1 -> Sum1/2, Sum6/1
  Discrete-Time Integrator/State -> Sum1/1
  Sum1/1 -> Relational Operator1/1, Relational Operator/1
  Logical Operator2/1 -> Switch/2
  Relational Operator/1 -> Logical Operator/1  "UpperLimit_is_Reached"
  Relational Operator1/1 -> Logical Operator1/1  "LowerLimit_Is_Reached"
  Constant1/1 -> Relational Operator/2
  Constant3/1 -> Relational Operator1/2
  Compare To Zero/1 -> Logical Operator/2  "Error_is_positive"
  Logical Operator/1 -> Logical Operator2/1
  Logical Operator1/1 -> Logical Operator2/2
  Compare To Zero1/1 -> Logical Operator1/2  "Error_is_negative"
  Error/1 -> Compare To Zero1/1, Compare To Zero/1, Kp4/1, Kp5/1
  Sum6/1 -> Saturation2/1
  Kp4/1 -> Zero-Order Hold/1
  Discrete-Time Integrator/1 -> Sum6/2
  Saturation2/1 -> Out/1
  Switch/1 -> Discrete-Time Integrator/1
  Kp5/1 -> Switch/3

== system lib_dGrid/MMC-configurable control modes/MMC Control/Compensation Modes & AC//DC to Arm transform Number of inserted (Nin) and blocked (Nbl) modules/PWM/PWM Gen1 ==
  Uref : Inport
  Add6 : Sum
  Clock1 : DigitalClock  SampleTime=Ts
  Data Type Conversion : DataTypeConversion  OutDataTypeStr=double  SaturateOnIntegerOverflow=off  RndMeth=Floor
  Fc1 : Constant  Value=Tc
  Fc2 : Constant  Value=Fc
  Logical Operator2 : Logic  Operator=NOT  AllPortsSameDT=off  OutDataTypeStr=boolean
  Lookup Table1 : Lookup  InputValues=[0 .5 1]  Table=[-1 1 -1]  LookUpMeth=Interpolation-Use End Values  SaturateOnIntegerOverflow=off
  Math Function1 : Math  Operator=rem  SignedPower=on
  Mux6 : Mux  Inputs=2
  Phase_rad1 : Constant  Value=Offset_Cr
  Product2 : Product  RndMeth=Zero
  Relational Operator1 : RelationalOperator  OutDataTypeStr=boolean
  SelectPulses : Selector  InputPortWidth=2*n  IndexOptions=Index vector (dialog)  Indices=SelectPulsesPS  OutputSizes=1
  P : Outport  VectorParamsAs1DForOutWhenUnconnected=off
  Cr : Outport  Port=2  VectorParamsAs1DForOutWhenUnconnected=off
  wires:
  Data Type Conversion/1 -> P/1
  SelectPulses/1 -> Data Type Conversion/1
  Uref/1 -> Relational Operator1/1
  Lookup Table1/1 -> Relational Operator1/2, Cr/1
  Phase_rad1/1 -> Add6/2
  Fc2/1 -> Product2/2
  Logical Operator2/1 -> Mux6/2
  Mux6/1 -> SelectPulses/1
  Fc1/1 -> Math Function1/2
  Clock1/1 -> Add6/1
  Add6/1 -> Math Function1/1
  Product2/1 -> Lookup Table1/1
  Relational Operator1/1 -> Logical Operator2/1, Mux6/1
  Math Function1/1 -> Product2/1

== system lib_dGrid/MMC-configurable control modes/MMC Control/Compensation Modes & AC//DC to Arm transform Number of inserted (Nin) and blocked (Nbl) modules/PWM/PWM Gen2 ==
  Uref : Inport
  Add6 : Sum
  Clock1 : DigitalClock  SampleTime=Ts
  Data Type Conversion : DataTypeConversion  OutDataTypeStr=double  SaturateOnIntegerOverflow=off  RndMeth=Floor
  Fc1 : Constant  Value=Tc
  Fc2 : Constant  Value=Fc
  Logical Operator2 : Logic  Operator=NOT  AllPortsSameDT=off  OutDataTypeStr=boolean
  Lookup Table1 : Lookup  InputValues=[0 .5 1]  Table=[-1 1 -1]  LookUpMeth=Interpolation-Use End Values  SaturateOnIntegerOverflow=off
  Math Function1 : Math  Operator=rem  SignedPower=on
  Mux6 : Mux  Inputs=2
  Phase_rad1 : Constant  Value=Offset_Cr
  Product2 : Product  RndMeth=Zero
  Relational Operator1 : RelationalOperator  OutDataTypeStr=boolean
  SelectPulses : Selector  InputPortWidth=2*n  IndexOptions=Index vector (dialog)  Indices=SelectPulsesPS  OutputSizes=1
  P : Outport  VectorParamsAs1DForOutWhenUnconnected=off
  Cr : Outport  Port=2  VectorParamsAs1DForOutWhenUnconnected=off
  wires:
  Math Function1/1 -> Product2/1
  Relational Operator1/1 -> Mux6/1, Logical Operator2/1
  Product2/1 -> Lookup Table1/1
  Add6/1 -> Math Function1/1
  Clock1/1 -> Add6/1
  Fc1/1 -> Math Function1/2
  Mux6/1 -> SelectPulses/1
  Logical Operator2/1 -> Mux6/2
  Fc2/1 -> Product2/2
  Phase_rad1/1 -> Add6/2
  Lookup Table1/1 -> Cr/1, Relational Operator1/2
  Uref/1 -> Relational Operator1/1
  SelectPulses/1 -> Data Type Conversion/1
  Data Type Conversion/1 -> P/1

== system lib_dGrid/MMC-configurable control modes/MMC Control/Compensation Modes & AC//DC to Arm transform Number of inserted (Nin) and blocked (Nbl) modules/PWM/PWM Gen3 ==
  Uref : Inport
  Add6 : Sum
  Clock1 : DigitalClock  SampleTime=Ts
  Data Type Conversion : DataTypeConversion  OutDataTypeStr=double  SaturateOnIntegerOverflow=off  RndMeth=Floor
  Fc1 : Constant  Value=Tc
  Fc2 : Constant  Value=Fc
  Logical Operator2 : Logic  Operator=NOT  AllPortsSameDT=off  OutDataTypeStr=boolean
  Lookup Table1 : Lookup  InputValues=[0 .5 1]  Table=[-1 1 -1]  LookUpMeth=Interpolation-Use End Values  SaturateOnIntegerOverflow=off
  Math Function1 : Math  Operator=rem  SignedPower=on
  Mux6 : Mux  Inputs=2
  Phase_rad1 : Constant  Value=Offset_Cr
  Product2 : Product  RndMeth=Zero
  Relational Operator1 : RelationalOperator  OutDataTypeStr=boolean
  SelectPulses : Selector  InputPortWidth=2*n  IndexOptions=Index vector (dialog)  Indices=SelectPulsesPS  OutputSizes=1
  P : Outport  VectorParamsAs1DForOutWhenUnconnected=off
  Cr : Outport  Port=2  VectorParamsAs1DForOutWhenUnconnected=off
  wires:
  Data Type Conversion/1 -> P/1
  SelectPulses/1 -> Data Type Conversion/1
  Uref/1 -> Relational Operator1/1
  Lookup Table1/1 -> Relational Operator1/2, Cr/1
  Phase_rad1/1 -> Add6/2
  Fc2/1 -> Product2/2
  Logical Operator2/1 -> Mux6/2
  Mux6/1 -> SelectPulses/1
  Fc1/1 -> Math Function1/2
  Clock1/1 -> Add6/1
  Add6/1 -> Math Function1/1
  Product2/1 -> Lookup Table1/1
  Relational Operator1/1 -> Logical Operator2/1, Mux6/1
  Math Function1/1 -> Product2/1

== system lib_dGrid/MMC-configurable control modes/MMC Control/Compensation Modes & AC//DC to Arm transform Number of inserted (Nin) and blocked (Nbl) modules/PWM/PWM Gen4 ==
  Uref : Inport
  Add6 : Sum
  Clock1 : DigitalClock  SampleTime=Ts
  Data Type Conversion : DataTypeConversion  OutDataTypeStr=double  SaturateOnIntegerOverflow=off  RndMeth=Floor
  Fc1 : Constant  Value=Tc
  Fc2 : Constant  Value=Fc
  Logical Operator2 : Logic  Operator=NOT  AllPortsSameDT=off  OutDataTypeStr=boolean
  Lookup Table1 : Lookup  InputValues=[0 .5 1]  Table=[-1 1 -1]  LookUpMeth=Interpolation-Use End Values  SaturateOnIntegerOverflow=off
  Math Function1 : Math  Operator=rem  SignedPower=on
  Mux6 : Mux  Inputs=2
  Phase_rad1 : Constant  Value=Offset_Cr
  Product2 : Product  RndMeth=Zero
  Relational Operator1 : RelationalOperator  OutDataTypeStr=boolean
  SelectPulses : Selector  InputPortWidth=2*n  IndexOptions=Index vector (dialog)  Indices=SelectPulsesPS  OutputSizes=1
  P : Outport  VectorParamsAs1DForOutWhenUnconnected=off
  Cr : Outport  Port=2  VectorParamsAs1DForOutWhenUnconnected=off
  wires:
  Math Function1/1 -> Product2/1
  Relational Operator1/1 -> Mux6/1, Logical Operator2/1
  Product2/1 -> Lookup Table1/1
  Add6/1 -> Math Function1/1
  Clock1/1 -> Add6/1
  Fc1/1 -> Math Function1/2
  Mux6/1 -> SelectPulses/1
  Logical Operator2/1 -> Mux6/2
  Fc2/1 -> Product2/2
  Phase_rad1/1 -> Add6/2
  Lookup Table1/1 -> Cr/1, Relational Operator1/2
  Uref/1 -> Relational Operator1/1
  SelectPulses/1 -> Data Type Conversion/1
  Data Type Conversion/1 -> P/1

== system lib_dGrid/MMC-configurable control modes/MMC Control/Compensation Modes & AC//DC to Arm transform Number of inserted (Nin) and blocked (Nbl) modules/PWM/PWM Gen5 ==
  Uref : Inport
  Add6 : Sum
  Clock1 : DigitalClock  SampleTime=Ts
  Data Type Conversion : DataTypeConversion  OutDataTypeStr=double  SaturateOnIntegerOverflow=off  RndMeth=Floor
  Fc1 : Constant  Value=Tc
  Fc2 : Constant  Value=Fc
  Logical Operator2 : Logic  Operator=NOT  AllPortsSameDT=off  OutDataTypeStr=boolean
  Lookup Table1 : Lookup  InputValues=[0 .5 1]  Table=[-1 1 -1]  LookUpMeth=Interpolation-Use End Values  SaturateOnIntegerOverflow=off
  Math Function1 : Math  Operator=rem  SignedPower=on
  Mux6 : Mux  Inputs=2
  Phase_rad1 : Constant  Value=Offset_Cr
  Product2 : Product  RndMeth=Zero
  Relational Operator1 : RelationalOperator  OutDataTypeStr=boolean
  SelectPulses : Selector  InputPortWidth=2*n  IndexOptions=Index vector (dialog)  Indices=SelectPulsesPS  OutputSizes=1
  P : Outport  VectorParamsAs1DForOutWhenUnconnected=off
  Cr : Outport  Port=2  VectorParamsAs1DForOutWhenUnconnected=off
  wires:
  Data Type Conversion/1 -> P/1
  SelectPulses/1 -> Data Type Conversion/1
  Uref/1 -> Relational Operator1/1
  Lookup Table1/1 -> Relational Operator1/2, Cr/1
  Phase_rad1/1 -> Add6/2
  Fc2/1 -> Product2/2
  Logical Operator2/1 -> Mux6/2
  Mux6/1 -> SelectPulses/1
  Fc1/1 -> Math Function1/2
  Clock1/1 -> Add6/1
  Add6/1 -> Math Function1/1
  Product2/1 -> Lookup Table1/1
  Relational Operator1/1 -> Logical Operator2/1, Mux6/1
  Math Function1/1 -> Product2/1

== system lib_dGrid/MMC-configurable control modes/MMC Control/Compensation Modes & AC//DC to Arm transform Number of inserted (Nin) and blocked (Nbl) modules/PWM/PWM Gen6 ==
  Uref : Inport
  Add6 : Sum
  Clock1 : DigitalClock  SampleTime=Ts
  Data Type Conversion : DataTypeConversion  OutDataTypeStr=double  SaturateOnIntegerOverflow=off  RndMeth=Floor
  Fc1 : Constant  Value=Tc
  Fc2 : Constant  Value=Fc
  Logical Operator2 : Logic  Operator=NOT  AllPortsSameDT=off  OutDataTypeStr=boolean
  Lookup Table1 : Lookup  InputValues=[0 .5 1]  Table=[-1 1 -1]  LookUpMeth=Interpolation-Use End Values  SaturateOnIntegerOverflow=off
  Math Function1 : Math  Operator=rem  SignedPower=on
  Mux6 : Mux  Inputs=2
  Phase_rad1 : Constant  Value=Offset_Cr
  Product2 : Product  RndMeth=Zero
  Relational Operator1 : RelationalOperator  OutDataTypeStr=boolean
  SelectPulses : Selector  InputPortWidth=2*n  IndexOptions=Index vector (dialog)  Indices=SelectPulsesPS  OutputSizes=1
  P : Outport  VectorParamsAs1DForOutWhenUnconnected=off
  Cr : Outport  Port=2  VectorParamsAs1DForOutWhenUnconnected=off
  wires:
  Math Function1/1 -> Product2/1
  Relational Operator1/1 -> Mux6/1, Logical Operator2/1
  Product2/1 -> Lookup Table1/1
  Add6/1 -> Math Function1/1
  Clock1/1 -> Add6/1
  Fc1/1 -> Math Function1/2
  Mux6/1 -> SelectPulses/1
  Logical Operator2/1 -> Mux6/2
  Fc2/1 -> Product2/2
  Phase_rad1/1 -> Add6/2
  Lookup Table1/1 -> Cr/1, Relational Operator1/2
  Uref/1 -> Relational Operator1/1
  SelectPulses/1 -> Data Type Conversion/1
  Data Type Conversion/1 -> P/1

== system lib_dGrid/MMC-configurable control modes/MMC Control/PLL, Measurements and Transformation/Symmetrical PLL/Angle Integrator [SI] ==
  omega : Inport
  phi0 : Inport  Port=2
  Bias : Bias  Bias=-2*pi  SaturateOnIntegerOverflow=off
  Bias1 : Bias  Bias=2*pi  SaturateOnIntegerOverflow=off
  Delay : Delay  DelayLength=1  InitialConditionSource=Input port  SampleTime=Ts
      settings: InputPortMap=u0,p4
  Gain3 : Gain  Gain=Ts
  Sum : Sum  Inputs=|++
  Switch : Switch  Criteria=u2 > Threshold  Threshold=pi  SaturateOnIntegerOverflow=off  InputSameDT=off
  Switch1 : Switch  Threshold=-pi  SaturateOnIntegerOverflow=off  InputSameDT=off
  phi : Outport  VectorParamsAs1DForOutWhenUnconnected=off
  wires:
  Switch1/1 -> Delay/1
  Bias1/1 -> Switch1/3
  Switch/1 -> Switch1/2, Bias1/1, Switch1/1
  Delay/1 -> phi/1, Sum/2
  Sum/1 -> Bias/1, Switch/2, Switch/3
  Bias/1 -> Switch/1
  Gain3/1 -> Sum/1
  omega/1 -> Gain3/1
  phi0/1 -> Delay/2

== system lib_dGrid/MMC-configurable control modes/MMC Control/PLL, Measurements and Transformation/Symmetrical PLL/PhN->ab0 ==
  PhN : Inport
  AlphaBetaNull Transformation : Gain  Gain="[2/3   -1/3    -1/3;   0   1/sqrt(3) -1/sqrt(3); 1/3 1/3 1/3]"  Multiplication=Matrix(K*u) (u vector)
  ab0 : Outport  VectorParamsAs1DForOutWhenUnconnected=off
  wires:
  AlphaBetaNull Transformation/1 -> ab0/1
  PhN/1 -> AlphaBetaNull Transformation/1

== system lib_dGrid/MMC-configurable control modes/MMC Control/PLL, Measurements and Transformation/Symmetrical PLL/ab0->dq0-faster ==
  ab0 : Inport
  w : Inport  Port=2
  Demux : Demux  Outputs=3
  Mux : Mux  Inputs=3
  Product{,1..3} (4 alike) : Product
  Subtract : Sum
  Subtract1 : Sum  Inputs=-+
  Trigonometric Function : Trigonometry  Operator=sincos
  dq0 : Outport  VectorParamsAs1DForOutWhenUnconnected=off
  wires:
  Subtract/1 -> Mux/1
  Subtract1/1 -> Mux/2
  Product3/1 -> Subtract1/2
  Product2/1 -> Subtract1/1
  Product1/1 -> Subtract/2
  Product/1 -> Subtract/1
  Trigonometric Function/1 -> Product1/1, Product2/1
  Trigonometric Function/2 -> Product3/1, Product/1
  Demux/2 -> Product3/2, Product1/2
  w/1 -> Trigonometric Function/1
  ab0/1 -> Demux/1
  Demux/1 -> Product/2, Product2/2
  Demux/3 -> Mux/3
  Mux/1 -> dq0/1

== system lib_dGrid/MMC-configurable control modes/MMC Control/PLL, Measurements and Transformation/Symmetrical PLL/discrete PID ==
  e : Inport
  Gain : Gain  Gain=Kp
  Gain1 : Gain  Gain=Ki*Ts
  Gain2 : Gain  Gain=Kd/Ts
  Sum1 : Sum  Inputs=+++
  Sum2 : Sum  Inputs=|++
  Sum3 : Sum  Inputs=|-+
  Unit Delay2 : UnitDelay  SampleTime=Ts  HasFrameUpgradeWarning=on
  Unit Delay3 : UnitDelay  InitialCondition=x_init  SampleTime=Ts  HasFrameUpgradeWarning=on
  y : Outport  VectorParamsAs1DForOutWhenUnconnected=off
  wires:
  e/1 -> Gain/1, Gain1/1, Unit Delay2/1, Sum3/1
  Unit Delay2/1 -> Sum3/2
  Sum1/1 -> y/1
  Gain/1 -> Sum1/1
  Unit Delay3/1 -> Sum1/2, Sum2/2
  Gain2/1 -> Sum1/3
  Gain1/1 -> Sum2/1
  Sum3/1 -> Gain2/1
  Sum2/1 -> Unit Delay3/1

== system lib_dGrid/MMC-configurable control modes/MMC Control/PLL, Measurements and Transformation/from DDSRF-PLL/PT1 as IIR ==
  U : Inport
  Gain : Gain  Gain=K*T/(T+2*tau)  SampleTime=T
  Gain1 : Gain  Gain=K*T/(T+2*tau)
  Gain2 : Gain  Gain=(T-2*tau)/(T+2*tau)
  Sum : Sum  Inputs=|++
  Sum1 : Sum  Inputs=+|-
  Unit Delay : UnitDelay  InitialCondition=Init  SampleTime=T  HasFrameUpgradeWarning=on
  Unit Delay1 : UnitDelay  InitialCondition=Init*K  SampleTime=T  HasFrameUpgradeWarning=on
  Y : Outport  VectorParamsAs1DForOutWhenUnconnected=off
  wires:
  Gain2/1 -> Sum1/2
  Sum1/1 -> Sum/2
  Gain1/1 -> Sum1/1
  Unit Delay1/1 -> Gain2/1
  Sum/1 -> Y/1, Unit Delay1/1
  Gain/1 -> Sum/1
  Unit Delay/1 -> Gain1/1
  U/1 -> Gain/1, Unit Delay/1
